simulink model "TestingModel"  (R2015a)
settings: Solver=ode3  StartTime=0.0  StopTime=10.0  FixedStep=0.0001  RelTol=1e-3
undefined symbols (not defined in the file or in its folder): sigbuilder_block
settings Model: CovSFcnEnable=off  Creator=HP  LastModifiedBy=adelgayed60
settings DebuggingCC: SolverPrmCheckMsg=warning

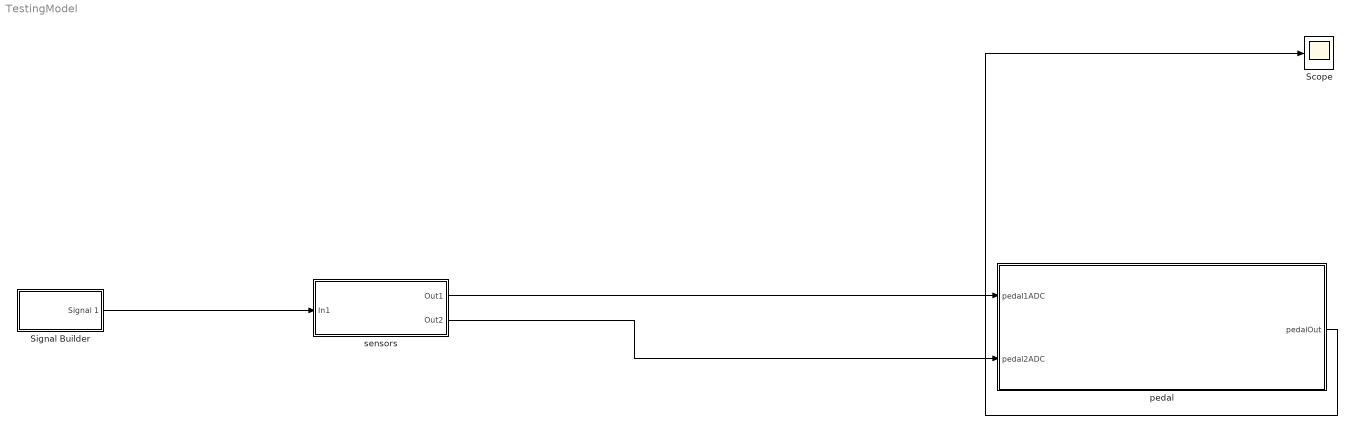
== system TestingModel ==
  Scope : Scope  NumInputPorts=3
      settings: YMin=-5~-5~-5  YMax=5~5~5
  Signal Builder : Subsystem  Tag=STV Subsys  LoadFcn=sigbuilder_block('load');  StartFcn=sigbuilder_block('start');  StopFcn=sigbuilder_block('stop');  ClipboardFcn=sigbuilder_block('clipboard');  mask(Sigbuilder block){}
      mask help: Simulink:masks:SigbuilderBlock_MD
      mask init:
      | if ~strcmp(get_param(bdroot(gcbh),'SimulationStatus'),'stopped') tuvar = sigbuilder_block('maskInit'); end
      settings: CopyFcn=sigbuilder_block('copy');  DeleteFcn=sigbuilder_block('delete');  ModelCloseFcn=sigbuilder_block('modelClose');  PreSaveFcn=sigbuilder_block('preSave');  PauseFcn=sigbuilder_block('pause');  ContinueFcn=sigbuilder_block('continue');  NameChangeFcn=sigbuilder_block('namechange');  OpenFcn=sigbuilder_block('open',[437.25 180 550.5 395.25 ]);  CloseFcn=sigbuilder_block('close');
      mask Display: plot(0, 0, 100, 100,[2, 2, 32, 32, 2], [68, 8, 8, 68, 68],[32, 2], [38, 38], [32, 19, 2],[53, 60, 44], [32, 17, 17, 2],[16, 16, 31, 31]);txt = getActiveGroup(gcbh);text(2, 100, txt,'verticalAlignment', 'top');
  pedal : Subsystem
  sensors : Subsystem
  wires:
  Signal Builder/1(Signal 1) -> sensors/1(In1)
  sensors/1(Out1) -> pedal/1(pedal1ADC)
  sensors/2(Out2) -> pedal/2(pedal2ADC)
  pedal/1(pedalOut) -> Scope/2

== system TestingModel/Signal Builder ==
  Demux : Demux  Tag=STV Demux  Outputs=1
  FromWs : FromWorkspace  Tag=STV FromWs  VariableName=tuvar  SampleTime=0
      SigBuilderData=|
      | common.afterFinalStr = 'Extrapolate'
      | common.sampleTime = 0
      | dataSet.timeRange = [0 10]
      | dataSet.name = 'Group 1'
      | sbobj.Groups.Name = 'Group 1'
      | sbobj.Groups.Signals.Name = 'Signal 1'
      | sbobj.Groups.Signals.XData = [0 10]
      | sbobj.Groups.Signals.YData = [-7 113]
  Signal 1 : Outport  Tag=STV Outport
  wires:
  Demux/1 -> Signal 1/1
  FromWs/1 -> Demux/1

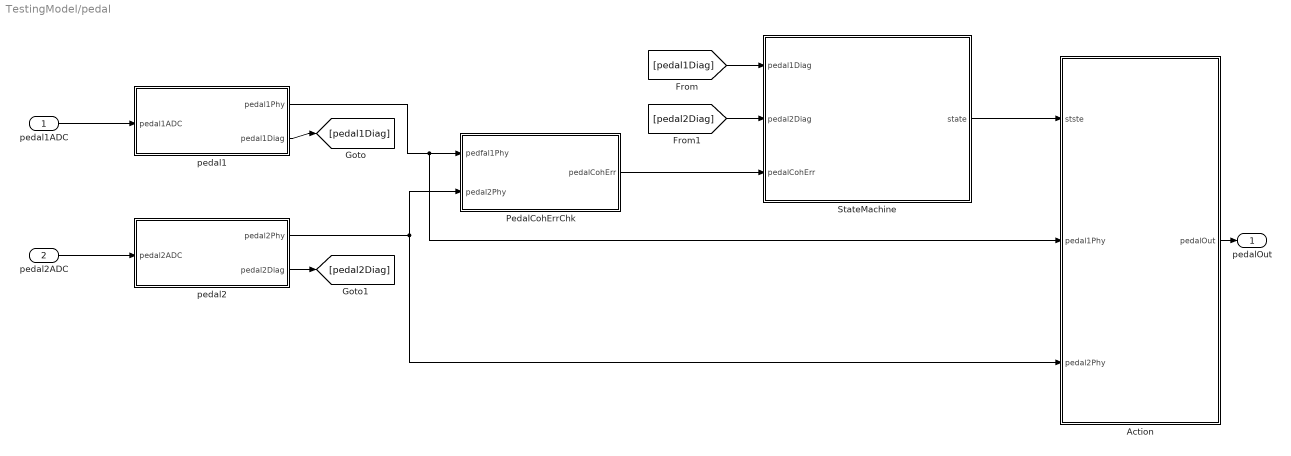
== system TestingModel/pedal ==
  pedal1ADC : Inport
  pedal2ADC : Inport  Port=2
  Action : Subsystem
  PedalCohErrChk : Subsystem
  StateMachine : Subsystem
  pedal1 : Subsystem
  pedal2 : Subsystem
  pedalOut : Outport
  wires:
  [pedal1Diag] -> StateMachine/1(pedal1Diag)
  PedalCohErrChk/1(pedalCohErr) -> StateMachine/3(pedalCohErr)
  pedal2/2(pedal2Diag) -> [pedal2Diag]
  pedal1/2(pedal1Diag) -> [pedal1Diag]
  [pedal2Diag] -> StateMachine/2(pedal2Diag)
  pedal1/1(pedal1Phy) -> Action/2(pedal1Phy), PedalCohErrChk/1(pedfal1Phy)
  pedal2/1(pedal2Phy) -> Action/3(pedal2Phy), PedalCohErrChk/2(pedal2Phy)
  pedal1ADC/1 -> pedal1/1(pedal1ADC)
  pedal2ADC/1 -> pedal2/1(pedal2ADC)
  Action/1(pedalOut) -> pedalOut/1
  StateMachine/1(state) -> Action/1(stste)

== system TestingModel/sensors ==
  In1 : Inport
  sensor1 : Subsystem
  sensor2 : Subsystem
  Out1 : Outport
  Out2 : Outport  Port=2
  wires:
  In1/1 -> sensor2/1(In1), sensor1/1(In1)
  sensor2/1(Out1) -> Out2/1
  sensor1/1(Out1) -> Out1/1

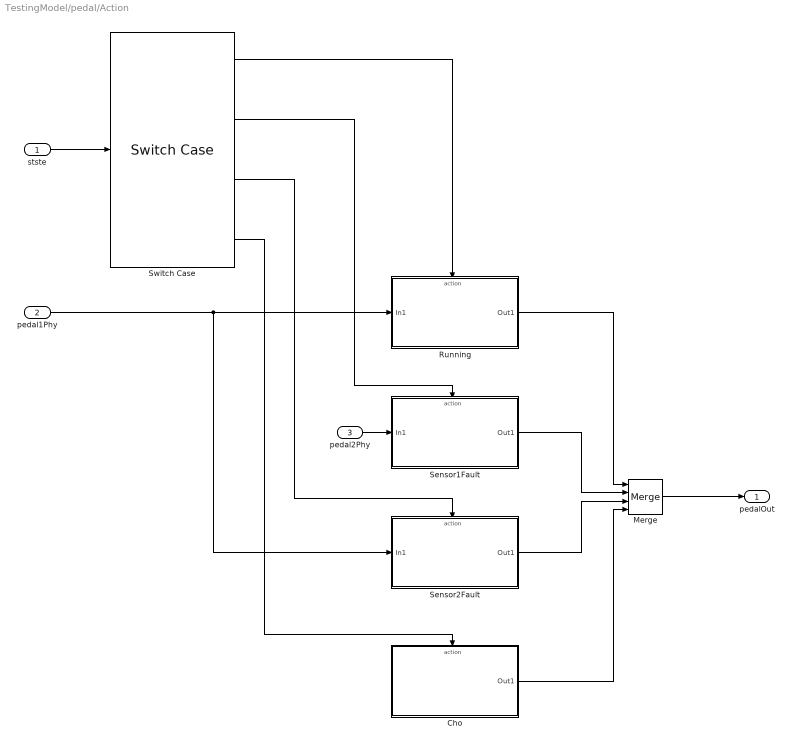
== system TestingModel/pedal/Action ==
  stste : Inport
  pedal1Phy : Inport  Port=2
  pedal2Phy : Inport  Port=3
  Cho : Subsystem  TreatAsAtomicUnit=on
  Merge : Merge  Inputs=4
  Running : Subsystem  TreatAsAtomicUnit=on
  Sensor1Fault : Subsystem  TreatAsAtomicUnit=on
  Sensor2Fault : Subsystem  TreatAsAtomicUnit=on
  Switch Case : SwitchCase  CaseConditions={0, 1, 2, 3}  ShowDefaultCase=off
  pedalOut : Outport
  wires:
  Switch Case/1 -> Running/Action
  Switch Case/2 -> Sensor1Fault/Action
  Switch Case/4 -> Cho/Action
  Switch Case/3 -> Sensor2Fault/Action
  stste/1 -> Switch Case/1
  Running/1(Out1) -> Merge/1
  Cho/1(Out1) -> Merge/4
  Sensor1Fault/1(Out1) -> Merge/2
  Sensor2Fault/1(Out1) -> Merge/3
  pedal2Phy/1 -> Sensor1Fault/1(In1)
  pedal1Phy/1 -> Sensor2Fault/1(In1), Running/1(In1)
  Merge/1 -> pedalOut/1

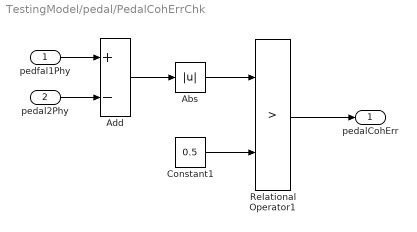
== system TestingModel/pedal/PedalCohErrChk ==
  pedfal1Phy : Inport
  pedal2Phy : Inport  Port=2
  Abs : Abs
  Add : Sum  Inputs=+-
  Constant1 : Constant  Value=0.5  OutDataTypeStr=single
  Relational Operator1 : RelationalOperator  Operator=>  OutDataTypeStr=boolean
  pedalCohErr : Outport
  wires:
  Relational Operator1/1 -> pedalCohErr/1
  pedfal1Phy/1 -> Add/1
  Add/1 -> Abs/1
  pedal2Phy/1 -> Add/2
  Constant1/1 -> Relational Operator1/2
  Abs/1 -> Relational Operator1/1

== system TestingModel/pedal/StateMachine ==
  pedal1Diag : Inport
  pedal2Diag : Inport  Port=2
  pedalCohErr : Inport  Port=3
  StateMachine : Stateflow chart  TreatAsAtomicUnit=on
  state : Outport
  wires:
  pedalCohErr/1 -> StateMachine/3(peddalCohErr)
  StateMachine/1(state) -> state/1
  pedal2Diag/1 -> StateMachine/2(pedal2Diag)
  pedal1Diag/1 -> StateMachine/1(pedal1Diag)

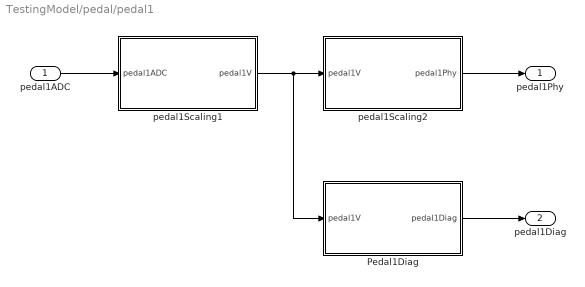
== system TestingModel/pedal/pedal1 ==
  pedal1ADC : Inport
  Pedal1Diag : Subsystem
  pedal1Scaling1 : Subsystem
  pedal1Scaling2 : Subsystem
  pedal1Phy : Outport
  pedal1Diag : Outport  Port=2
  wires:
  pedal1Scaling1/1(pedal1V) -> pedal1Scaling2/1(pedal1V), Pedal1Diag/1(pedal1V)
  pedal1Scaling2/1(pedal1Phy) -> pedal1Phy/1
  Pedal1Diag/1(pedal1Diag) -> pedal1Diag/1
  pedal1ADC/1 -> pedal1Scaling1/1(pedal1ADC)

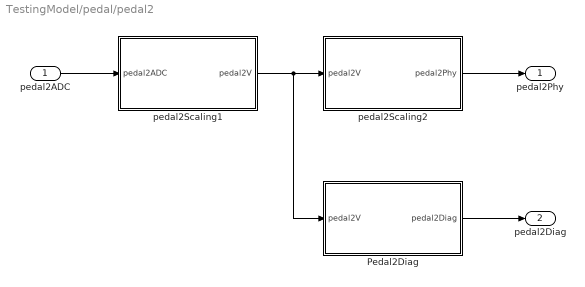
== system TestingModel/pedal/pedal2 ==
  pedal2ADC : Inport
  Pedal2Diag : Subsystem
  pedal2Scaling1 : Subsystem
  pedal2Scaling2 : Subsystem
  pedal2Phy : Outport
  pedal2Diag : Outport  Port=2
  wires:
  pedal2ADC/1 -> pedal2Scaling1/1(pedal2ADC)
  Pedal2Diag/1(pedal2Diag) -> pedal2Diag/1
  pedal2Scaling2/1(pedal2Phy) -> pedal2Phy/1
  pedal2Scaling1/1(pedal2V) -> Pedal2Diag/1(pedal2V), pedal2Scaling2/1(pedal2V)

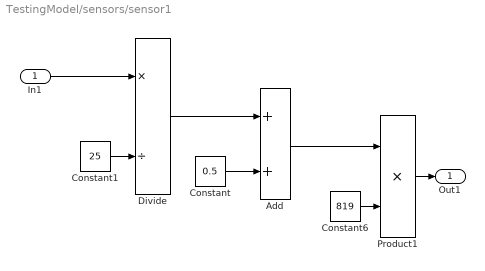
== system TestingModel/sensors/sensor1 ==
  In1 : Inport
  Add : Sum
  Constant : Constant  Value=0.5  OutDataTypeStr=single
  Constant1 : Constant  Value=25  OutDataTypeStr=single
  Constant6 : Constant  Value=819  OutDataTypeStr=single
  Divide : Product  Inputs=*/
  Product1 : Product  OutDataTypeStr=uint16
  Out1 : Outport
  wires:
  Constant6/1 -> Product1/2
  Add/1 -> Product1/1
  Product1/1 -> Out1/1
  In1/1 -> Divide/1
  Constant/1 -> Add/2
  Constant1/1 -> Divide/2
  Divide/1 -> Add/1

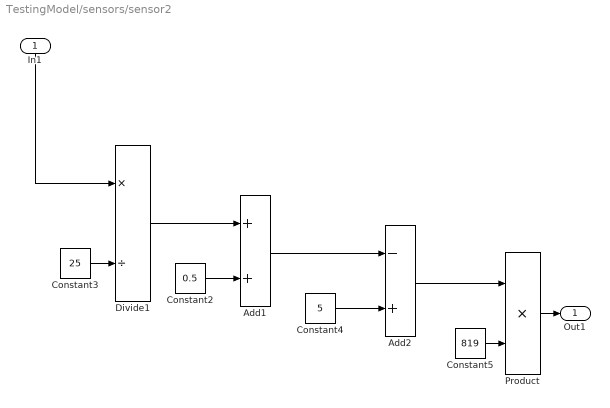
== system TestingModel/sensors/sensor2 ==
  In1 : Inport
  Add1 : Sum
  Add2 : Sum  Inputs=-+
  Constant2 : Constant  Value=0.5  OutDataTypeStr=single
  Constant3 : Constant  Value=25  OutDataTypeStr=single
  Constant4 : Constant  Value=5  OutDataTypeStr=single
  Constant5 : Constant  Value=819  OutDataTypeStr=single
  Divide1 : Product  Inputs=*/
  Product : Product  OutDataTypeStr=uint16
  Out1 : Outport
  wires:
  Add1/1 -> Add2/1
  Constant4/1 -> Add2/2
  Constant5/1 -> Product/2
  Product/1 -> Out1/1
  In1/1 -> Divide1/1
  Add2/1 -> Product/1
  Constant2/1 -> Add1/2
  Divide1/1 -> Add1/1
  Constant3/1 -> Divide1/2

== system TestingModel/pedal/Action/Cho ==
  Action Port : ActionPort  ActionType=case
  Constant1 : Constant  Value=0  OutDataTypeStr=single
  Out1 : Outport
  wires:
  Constant1/1 -> Out1/1

== system TestingModel/pedal/Action/Running ==
  In1 : Inport
  Action Port : ActionPort  ActionType=case
  Out1 : Outport
  wires:
  In1/1 -> Out1/1

== system TestingModel/pedal/Action/Sensor1Fault ==
  In1 : Inport
  Action Port : ActionPort  ActionType=case
  Saturation : Saturate  UpperLimit=20  LowerLimit=0
  Out1 : Outport
  wires:
  In1/1 -> Saturation/1
  Saturation/1 -> Out1/1

== system TestingModel/pedal/Action/Sensor2Fault ==
  In1 : Inport
  Action Port : ActionPort  ActionType=case
  Saturation : Saturate  UpperLimit=20  LowerLimit=0
  Out1 : Outport
  wires:
  Saturation/1 -> Out1/1
  In1/1 -> Saturation/1

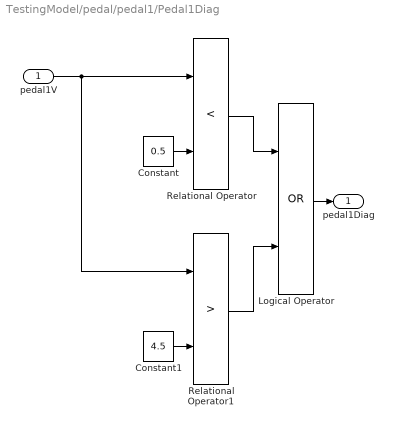
== system TestingModel/pedal/pedal1/Pedal1Diag ==
  pedal1V : Inport
  Constant : Constant  Value=0.5  OutDataTypeStr=single
  Constant1 : Constant  Value=4.5  OutDataTypeStr=single
  Logical Operator : Logic  Operator=OR  AllPortsSameDT=off  OutDataTypeStr=boolean
  Relational Operator : RelationalOperator  Operator=<  OutDataTypeStr=boolean
  Relational Operator1 : RelationalOperator  Operator=>  OutDataTypeStr=boolean
  pedal1Diag : Outport
  wires:
  Logical Operator/1 -> pedal1Diag/1
  Relational Operator/1 -> Logical Operator/1
  Constant1/1 -> Relational Operator1/2
  pedal1V/1 -> Relational Operator1/1, Relational Operator/1
  Relational Operator1/1 -> Logical Operator/2
  Constant/1 -> Relational Operator/2

== system TestingModel/pedal/pedal1/pedal1Scaling1 ==
  pedal1ADC : Inport
  Constant : Constant  Value=819  OutDataTypeStr=uint16
  Divide : Product  Inputs=*/  OutDataTypeStr=single
  Saturation : Saturate  UpperLimit=4095  LowerLimit=0  OutDataTypeStr=uint16
  pedal1V : Outport
  wires:
  Constant/1 -> Divide/2
  Divide/1 -> pedal1V/1
  pedal1ADC/1 -> Saturation/1
  Saturation/1 -> Divide/1

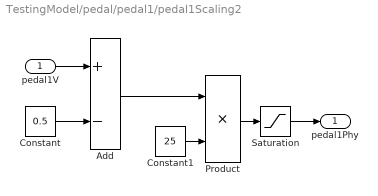
== system TestingModel/pedal/pedal1/pedal1Scaling2 ==
  pedal1V : Inport
  Add : Sum  Inputs=+-
  Constant : Constant  Value=0.5  OutDataTypeStr=single
  Constant1 : Constant  Value=25  OutDataTypeStr=single
  Product : Product
  Saturation : Saturate  UpperLimit=100  LowerLimit=0  OutDataTypeStr=single
  pedal1Phy : Outport
  wires:
  Constant/1 -> Add/2
  pedal1V/1 -> Add/1
  Constant1/1 -> Product/2
  Product/1 -> Saturation/1
  Add/1 -> Product/1
  Saturation/1 -> pedal1Phy/1

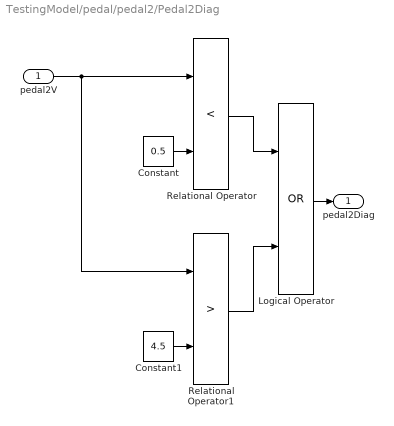
== system TestingModel/pedal/pedal2/Pedal2Diag ==
  pedal2V : Inport
  Constant : Constant  Value=0.5  OutDataTypeStr=single
  Constant1 : Constant  Value=4.5  OutDataTypeStr=single
  Logical Operator : Logic  Operator=OR  AllPortsSameDT=off  OutDataTypeStr=boolean
  Relational Operator : RelationalOperator  Operator=<  OutDataTypeStr=boolean
  Relational Operator1 : RelationalOperator  Operator=>  OutDataTypeStr=boolean
  pedal2Diag : Outport
  wires:
  Constant/1 -> Relational Operator/2
  Relational Operator1/1 -> Logical Operator/2
  pedal2V/1 -> Relational Operator/1, Relational Operator1/1
  Constant1/1 -> Relational Operator1/2
  Relational Operator/1 -> Logical Operator/1
  Logical Operator/1 -> pedal2Diag/1

== system TestingModel/pedal/pedal2/pedal2Scaling1 ==
  pedal2ADC : Inport
  Constant : Constant  Value=819  OutDataTypeStr=uint16
  Divide : Product  Inputs=*/  OutDataTypeStr=single
  Saturation : Saturate  UpperLimit=4095  LowerLimit=0  OutDataTypeStr=uint16
  pedal2V : Outport
  wires:
  Saturation/1 -> Divide/1
  pedal2ADC/1 -> Saturation/1
  Divide/1 -> pedal2V/1
  Constant/1 -> Divide/2

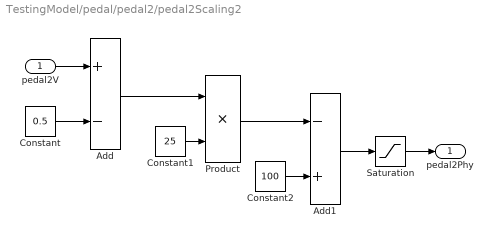
== system TestingModel/pedal/pedal2/pedal2Scaling2 ==
  pedal2V : Inport
  Add : Sum  Inputs=+-
  Add1 : Sum  Inputs=-+
  Constant : Constant  Value=0.5  OutDataTypeStr=single
  Constant1 : Constant  Value=25  OutDataTypeStr=single
  Constant2 : Constant  Value=100  OutDataTypeStr=single
  Product : Product
  Saturation : Saturate  UpperLimit=100  LowerLimit=0  OutDataTypeStr=single
  pedal2Phy : Outport
  wires:
  Saturation/1 -> pedal2Phy/1
  Add/1 -> Product/1
  Constant1/1 -> Product/2
  pedal2V/1 -> Add/1
  Constant/1 -> Add/2
  Product/1 -> Add1/1
  Constant2/1 -> Add1/2
  Add1/1 -> Saturation/1

== stateflow chart TestingModel/pedal/StateMachine/StateMachine ==
  state Running
    entry: state = uint8(0);
  state Sensor2Fault
    entry: state = uint8(2);
  state Sensor1Fault
    entry: state = uint8(1);
  state COH
    entry: state = uint8(3);
  (default) -> Running
  (junction 6) -> Running [order 5]
  Running -> (junction 6)
  (junction 6) -> Sensor2Fault [order 3] : [pedal2Diag]
  (junction 6) -> Sensor1Fault [order 2] : [pedal1Diag]
  Sensor2Fault -> (junction 6)
  Sensor1Fault -> (junction 6)
  (junction 6) -> COH [order 4] : [peddalCohErr]
  (junction 6) -> COH [order 1] : [pedal1Diag&&pedal2Diag]
  COH -> (junction 6)
  data: pedal1Diag input boolean size=1 [0..1]; pedal2Diag input boolean size=1 [0..1]; peddalCohErr input boolean size=1 [0..1]; state output uint8 size=1 [0..5]
